simulink model "LKAS_AutoSave_DF_20220414_1924_SW62"  (R2018b)
settings: Solver=FixedStepDiscrete  StartTime=0.0  StopTime=10.0  FixedStep=0.01  RelTol=1e-3
model workspace (MAT data in the model file):
  MCOS : class17 (value not decoded)
  MCOS : class17 (value not decoded)
  MCOS : class17 (value not decoded)
  MCOS : class17 (value not decoded)
  MCOS : class17 (value not decoded)
  MCOS : class17 (value not decoded)
  MCOS : class17 (value not decoded)
  MCOS : class17 (value not decoded)
  MCOS : class17 (value not decoded)
  MCOS : class17 (value not decoded)
  MCOS : class17 (value not decoded)
  MCOS : class17 (value not decoded)
  MCOS : class17 (value not decoded)
  MCOS : class17 (value not decoded)
  MCOS : class17 (value not decoded)
  MCOS : class17 (value not decoded)
  MCOS : class17 (value not decoded)
  MCOS : class17 (value not decoded)
  MCOS : class17 (value not decoded)
  MCOS : class17 (value not decoded)
  MCOS : class17 (value not decoded)
  MCOS : class17 (value not decoded)
  MCOS : class17 (value not decoded)
  MCOS : class17 (value not decoded)
  MCOS : class17 (value not decoded)
  MCOS : class17 (value not decoded)
  MCOS : class17 (value not decoded)
  MCOS : class17 (value not decoded)
  MCOS : class17 (value not decoded)
  MCOS : class17 (value not decoded)
  MCOS : class17 (value not decoded)
  MCOS : class17 (value not decoded)
  MCOS : class17 (value not decoded)
  MCOS : class17 (value not decoded)
  MCOS : class17 (value not decoded)
  MCOS : class17 (value not decoded)
  MCOS : class17 (value not decoded)
  MCOS : class17 (value not decoded)
  MCOS : class17 (value not decoded)
  MCOS : class17 (value not decoded)
  MCOS : class17 (value not decoded)
  MCOS : class17 (value not decoded)
  MCOS : class17 (value not decoded)
  MCOS : class17 (value not decoded)
  MCOS : class17 (value not decoded)
  MCOS : class17 (value not decoded)
  MCOS : class17 (value not decoded)
  MCOS : class17 (value not decoded)
  MCOS : class17 (value not decoded)
  MCOS : class17 (value not decoded)
  MCOS : class17 (value not decoded)
  MCOS : class17 (value not decoded)
  MCOS : class17 (value not decoded)
  MCOS : class17 (value not decoded)
  MCOS : class17 (value not decoded)
  MCOS : class17 (value not decoded)
  MCOS : class17 (value not decoded)
  MCOS : class17 (value not decoded)
  MCOS : class17 (value not decoded)
  MCOS : class17 (value not decoded)
  MCOS : class17 (value not decoded)
  MCOS : class17 (value not decoded)
  MCOS : class17 (value not decoded)
  MCOS : class17 (value not decoded)
  MCOS : class17 (value not decoded)
  MCOS : class17 (value not decoded)
  MCOS : class17 (value not decoded)
  MCOS : class17 (value not decoded)
  MCOS : class17 (value not decoded)
  MCOS : class17 (value not decoded)
  MCOS : class17 (value not decoded)
  MCOS : class17 (value not decoded)
  MCOS : class17 (value not decoded)
  MCOS : class17 (value not decoded)
  MCOS : class17 (value not decoded)
  MCOS : class17 (value not decoded)
  MCOS : class17 (value not decoded)
  MCOS : class17 (value not decoded)
  MCOS : class17 (value not decoded)
  MCOS : class17 (value not decoded)
  MCOS : class17 (value not decoded)
  MCOS : class17 (value not decoded)
  MCOS : class17 (value not decoded)
  MCOS : class17 (value not decoded)
  MCOS : class17 (value not decoded)
  MCOS : class17 (value not decoded)
  MCOS : class17 (value not decoded)
  MCOS : class17 (value not decoded)
  MCOS : class17 (value not decoded)
  MCOS : class17 (value not decoded)
  MCOS : class17 (value not decoded)
  MCOS : class17 (value not decoded)
  MCOS : class17 (value not decoded)
  MCOS : class17 (value not decoded)
  MCOS : class17 (value not decoded)
  MCOS : class17 (value not decoded)
  MCOS : class17 (value not decoded)
  MCOS : class17 (value not decoded)
  MCOS : class17 (value not decoded)
  MCOS : class17 (value not decoded)
  MCOS : class17 (value not decoded)
  MCOS : class17 (value not decoded)
  MCOS : class17 (value not decoded)
  MCOS : class17 (value not decoded)
  MCOS : class17 (value not decoded)
  MCOS : class17 (value not decoded)
  MCOS : class17 (value not decoded)
  MCOS : class17 (value not decoded)
  MCOS : class17 (value not decoded)
undefined symbols (not defined in the file): LKA_CarWidth, LKA_SampleTime, LKA_StrRatio_C, LKA_Veh2CamL_C, LKA_Veh2CamW_C, LKA_WhlBaseL_C, LL_CompHdAg_C, LL_CompSWA_C, LL_CrvtPrvwT_C, LL_DesDvt_C, LL_DvtComp_C, LL_DvtPrvwT_C, LL_DvtSpdDet_vDvtSpdMin_C, LL_HandsOff_ExitTime, LL_HandsOff_TextTime, LL_HandsOff_WarnTime, LL_HdAgExT_C, LL_HdAgPrvwT_C, LL_LAccMax_C, LL_LAccRMax_C, LL_LDW_EarliestWarnLine_C, LL_LDW_LatestWarnLine_C, LL_LDWS_SUPPRESS_HEADING, LL_LFClb_TFC_FfCtlRatio_C, LL_LFClb_TFC_KdBalance_C, LL_LFClb_TFC_KdMaxSWA_C, LL_LFClb_TFC_KdV1_C, LL_LFClb_TFC_KdV2_C, LL_LFClb_TFC_KdVehSpdLwr_C, LL_LFClb_TFC_KdVehSpdUpr_C, LL_LFClb_TFC_Ki_C, LL_LFClb_TFC_KiMaxSWA_C, LL_LFClb_TFC_Kp_C, LL_LFClb_TFC_KpKlat_C, LL_LFClb_TFC_KpV1_C, LL_LFClb_TFC_KpV2_C, LL_LFClb_TFC_KpVehSpdLwr_C, LL_LFClb_TFC_KpVehSpdUpr_C, LL_LFClb_TFC_PrvwT_C, LL_LKA_EarliestWarnLine_C, LL_LKA_EnableLine_DvtMax, LL_LKA_EnableLine_DvtMin, LL_LKA_EnableLine_Max, LL_LKA_LatestWarnLine_C, LL_LKAExPrcs_ExitC0Dvt, LL_LKAExPrcs_ExitC0Swt, LL_LKAExPrcs_tiExitDelayTime3, LL_LKAExPrcs_tiExitTime1, LL_LKAExPrcs_tiExitTime2, LL_LKAExPrcs_tiExitTime3, LL_LKAS_OUT_OF_CONTROL_LAT_VEL, LL_LKAS_OUT_OF_CONTROL_TTLC, LL_LKASWASyn_M0, LL_LKASWASyn_M1, LL_LKASWASyn_M2, LL_LKASWASyn_M3D, LL_LKASWASyn_M3K_DT, LL_LKASWASyn_M3K_MSD, LL_LKASWASyn_M4K, LL_LKASWASyn_SWAaddMax ... (+50)
libraries: simulink x234, canmsglib x6, dspstat3 x3, simulink_extras x1
(part 5 of 17)

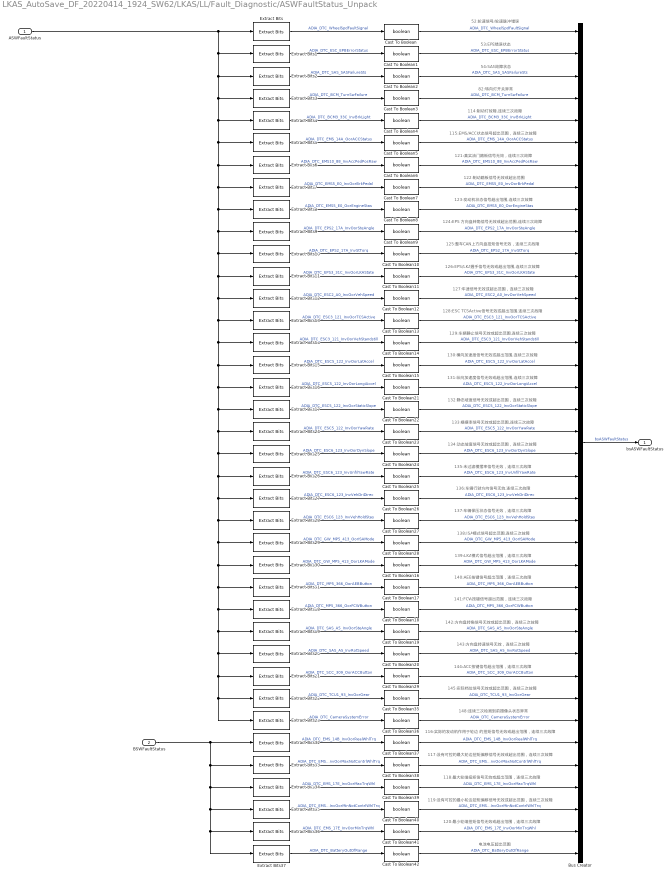
== system LKAS_AutoSave_DF_20220414_1924_SW62/LKAS/LL/Fault_Diagnostic/ASWFaultStatus_Unpack ==
  note: 117:没有可控的最大轮边扭矩偏移信号无效或超出范围，连续三次故障
  note: 120:最小轮端扭矩信号无效或超出范围，连续三次故障
  note: 116:实际的发动机作用于轮边 的扭矩信号无效或超出范围，连续三次故障
  note: 119:没有可控的最小轮边扭矩偏移信号无效或超出范围，连续三次故障
  note: 118:最大轮端扭矩信号无效或超出范围，连续三次故障
  note: 电池电压超出范围
  note: 148:连续三次检测到前摄像头状态异常
  note: 143:方向盘转速信号无效，连续三次故障
  note: 144:ACC按键信号超出范围，连续三次故障
  note: 145:实际档位信号无效或超出范围，连续三次故障
  note: 54:SAS故障状态
  note: 142:方向盘转角信号无效或超出范围，连续三次故障
  note: 121:真实油门踏板信号无效，连续三次故障
  note: 137:车辆保压状态信号无效，连续三次故障
  note: 114:制动灯故障,连续三次故障
  note: 115:EMS/ACC状态信号超出范围，连续三次故障
  note: 139:LKA模式信号超出范围，连续三次故障
  note: 53:EPB错误状态
  note: 123:发动机状态信号超出范围,连续三次故障
  note: 122:制动踏板信号无效或超出范围
  note: 124:EPS 方向盘转角信号无效或超出范围,连续三次故障
  note: 82:转向灯开关异常
  note: 52:轮速信号/轮速脉冲错误
  note: 130:横向加速度信号无效或超出范围,连续三次故障
  note: 134:动态坡度信号无效或超出范围，连续三次故障
  note: 131:纵向加速度信号无效或超出范围,连续三次故障
  note: 129:车辆静止信号无效或超出范围,连续三次故障
  note: 140:AEB按键信号超出范围，连续三次故障
  note: 128:ESC TCSActive信号无效或超出范围,连续三次故障
  note: 126:EPS/LKA握手信号无效或超出范围,连续三次故障
  note: 125:整车CAN上方向盘扭矩信号无效，连续三次故障
  note: 127:车速信号无效或超出范围，连续三次故障
  note: 141:FCW按键信号超出范围，连续三次故障
  note: 136:车辆行驶方向信号无效,连续三次故障
  note: 138:ISA模式信号超出范围,连续三次故障
  note: 135:未过滤横摆率信号无效，连续三次故障
  note: 133:横摆率信号无效或超出范围,连续三次故障
  note: 132:静态坡度信号无效或超出范围，连续三次故障
  ASWFaultStatus : Inport
  BSWFaultStatus : Inport  Port=2
  Bus Creator : BusCreator  Inputs=38
  Cast To Boolean{,1..29,35..42} (38 alike) : DataTypeConversion  OutDataTypeStr=boolean
  Extract Bits : simulink/Logic and Bit Operations/Extract Bits  bitsToExtract=Range of bits  numBits=8  bitIdxRange=0  outScalingMode=Preserve fixed-point scaling
      settings: SourceProductName=Simulink
  Extract Bits1 : simulink/Logic and Bit Operations/Extract Bits  bitsToExtract=Range of bits  numBits=8  bitIdxRange=1  outScalingMode=Treat bit field as an integer
      settings: SourceProductName=Simulink
  Extract Bits10 : simulink/Logic and Bit Operations/Extract Bits  bitsToExtract=Range of bits  numBits=8  bitIdxRange=10  outScalingMode=Treat bit field as an integer
      settings: SourceProductName=Simulink
  Extract Bits11 : simulink/Logic and Bit Operations/Extract Bits  bitsToExtract=Range of bits  numBits=8  bitIdxRange=11  outScalingMode=Treat bit field as an integer
      settings: SourceProductName=Simulink
  Extract Bits12 : simulink/Logic and Bit Operations/Extract Bits  bitsToExtract=Range of bits  numBits=8  bitIdxRange=12  outScalingMode=Treat bit field as an integer
      settings: SourceProductName=Simulink
  Extract Bits13 : simulink/Logic and Bit Operations/Extract Bits  bitsToExtract=Range of bits  numBits=8  bitIdxRange=13  outScalingMode=Treat bit field as an integer
      settings: SourceProductName=Simulink
  Extract Bits14 : simulink/Logic and Bit Operations/Extract Bits  bitsToExtract=Range of bits  numBits=8  bitIdxRange=14  outScalingMode=Treat bit field as an integer
      settings: SourceProductName=Simulink
  Extract Bits15 : simulink/Logic and Bit Operations/Extract Bits  bitsToExtract=Range of bits  numBits=8  bitIdxRange=15  outScalingMode=Treat bit field as an integer
      settings: SourceProductName=Simulink
  Extract Bits16 : simulink/Logic and Bit Operations/Extract Bits  bitsToExtract=Range of bits  numBits=8  bitIdxRange=16  outScalingMode=Treat bit field as an integer
      settings: SourceProductName=Simulink
  Extract Bits17 : simulink/Logic and Bit Operations/Extract Bits  bitsToExtract=Range of bits  numBits=8  bitIdxRange=17  outScalingMode=Treat bit field as an integer
      settings: SourceProductName=Simulink
  Extract Bits18 : simulink/Logic and Bit Operations/Extract Bits  bitsToExtract=Range of bits  numBits=8  bitIdxRange=26  outScalingMode=Treat bit field as an integer
      settings: SourceProductName=Simulink
  Extract Bits19 : simulink/Logic and Bit Operations/Extract Bits  bitsToExtract=Range of bits  numBits=8  bitIdxRange=27  outScalingMode=Treat bit field as an integer
      settings: SourceProductName=Simulink
  Extract Bits2 : simulink/Logic and Bit Operations/Extract Bits  bitsToExtract=Range of bits  numBits=8  bitIdxRange=2  outScalingMode=Treat bit field as an integer
      settings: SourceProductName=Simulink
  Extract Bits20 : simulink/Logic and Bit Operations/Extract Bits  bitsToExtract=Range of bits  numBits=8  bitIdxRange=28  outScalingMode=Treat bit field as an integer
      settings: SourceProductName=Simulink
  Extract Bits21 : simulink/Logic and Bit Operations/Extract Bits  bitsToExtract=Range of bits  numBits=8  bitIdxRange=29  outScalingMode=Treat bit field as an integer
      settings: SourceProductName=Simulink
  Extract Bits22 : simulink/Logic and Bit Operations/Extract Bits  bitsToExtract=Range of bits  numBits=8  bitIdxRange=30  outScalingMode=Treat bit field as an integer
      settings: SourceProductName=Simulink
  Extract Bits23 : simulink/Logic and Bit Operations/Extract Bits  bitsToExtract=Range of bits  numBits=8  bitIdxRange=31  outScalingMode=Treat bit field as an integer
      settings: SourceProductName=Simulink
  Extract Bits24 : simulink/Logic and Bit Operations/Extract Bits  bitsToExtract=Range of bits  numBits=8  bitIdxRange=18  outScalingMode=Treat bit field as an integer
      settings: SourceProductName=Simulink
  Extract Bits25 : simulink/Logic and Bit Operations/Extract Bits  bitsToExtract=Range of bits  numBits=8  bitIdxRange=19  outScalingMode=Treat bit field as an integer
      settings: SourceProductName=Simulink
  Extract Bits26 : simulink/Logic and Bit Operations/Extract Bits  bitsToExtract=Range of bits  numBits=8  bitIdxRange=20  outScalingMode=Treat bit field as an integer
      settings: SourceProductName=Simulink
  Extract Bits27 : simulink/Logic and Bit Operations/Extract Bits  bitsToExtract=Range of bits  numBits=8  bitIdxRange=21  outScalingMode=Treat bit field as an integer
      settings: SourceProductName=Simulink
  Extract Bits28 : simulink/Logic and Bit Operations/Extract Bits  bitsToExtract=Range of bits  numBits=8  bitIdxRange=22  outScalingMode=Treat bit field as an integer
      settings: SourceProductName=Simulink
  Extract Bits29 : simulink/Logic and Bit Operations/Extract Bits  bitsToExtract=Range of bits  numBits=8  bitIdxRange=23  outScalingMode=Treat bit field as an integer
      settings: SourceProductName=Simulink
  Extract Bits3 : simulink/Logic and Bit Operations/Extract Bits  bitsToExtract=Range of bits  numBits=8  bitIdxRange=3  outScalingMode=Treat bit field as an integer
      settings: SourceProductName=Simulink
  Extract Bits30 : simulink/Logic and Bit Operations/Extract Bits  bitsToExtract=Range of bits  numBits=8  bitIdxRange=24  outScalingMode=Treat bit field as an integer
      settings: SourceProductName=Simulink
  Extract Bits31 : simulink/Logic and Bit Operations/Extract Bits  bitsToExtract=Range of bits  numBits=8  bitIdxRange=25  outScalingMode=Treat bit field as an integer
      settings: SourceProductName=Simulink
  Extract Bits32 : simulink/Logic and Bit Operations/Extract Bits  bitsToExtract=Range of bits  numBits=8  bitIdxRange=26  outScalingMode=Treat bit field as an integer
      settings: SourceProductName=Simulink
  Extract Bits33 : simulink/Logic and Bit Operations/Extract Bits  bitsToExtract=Range of bits  numBits=8  bitIdxRange=27  outScalingMode=Treat bit field as an integer
      settings: SourceProductName=Simulink
  Extract Bits34 : simulink/Logic and Bit Operations/Extract Bits  bitsToExtract=Range of bits  numBits=8  bitIdxRange=28  outScalingMode=Treat bit field as an integer
      settings: SourceProductName=Simulink
  Extract Bits35 : simulink/Logic and Bit Operations/Extract Bits  bitsToExtract=Range of bits  numBits=8  bitIdxRange=29  outScalingMode=Treat bit field as an integer
      settings: SourceProductName=Simulink
  Extract Bits36 : simulink/Logic and Bit Operations/Extract Bits  bitsToExtract=Range of bits  numBits=8  bitIdxRange=30  outScalingMode=Treat bit field as an integer
      settings: SourceProductName=Simulink
  Extract Bits37 : simulink/Logic and Bit Operations/Extract Bits  bitsToExtract=Range of bits  numBits=8  bitIdxRange=31  outScalingMode=Treat bit field as an integer
      settings: SourceProductName=Simulink
  Extract Bits4 : simulink/Logic and Bit Operations/Extract Bits  bitsToExtract=Range of bits  numBits=8  bitIdxRange=4  outScalingMode=Treat bit field as an integer
      settings: SourceProductName=Simulink
  Extract Bits5 : simulink/Logic and Bit Operations/Extract Bits  bitsToExtract=Range of bits  numBits=8  bitIdxRange=5  outScalingMode=Treat bit field as an integer
      settings: SourceProductName=Simulink
  Extract Bits6 : simulink/Logic and Bit Operations/Extract Bits  bitsToExtract=Range of bits  numBits=8  bitIdxRange=6  outScalingMode=Treat bit field as an integer
      settings: SourceProductName=Simulink
  Extract Bits7 : simulink/Logic and Bit Operations/Extract Bits  bitsToExtract=Range of bits  numBits=8  bitIdxRange=7  outScalingMode=Treat bit field as an integer
      settings: SourceProductName=Simulink
  Extract Bits8 : simulink/Logic and Bit Operations/Extract Bits  bitsToExtract=Range of bits  numBits=8  bitIdxRange=8  outScalingMode=Treat bit field as an integer
      settings: SourceProductName=Simulink
  Extract Bits9 : simulink/Logic and Bit Operations/Extract Bits  bitsToExtract=Range of bits  numBits=8  bitIdxRange=9  outScalingMode=Treat bit field as an integer
      settings: SourceProductName=Simulink
  bsASWFaultStatus : Outport
  wires:
  Extract Bits37/1 -> Cast To Boolean42/1  "ADIA_DTC_BatteryOutOfRange"
  Extract Bits36/1 -> Cast To Boolean41/1  "ADIA_DTC_EMS_17E_InvOorMinTrqWhl"
  Extract Bits35/1 -> Cast To Boolean40/1  "ADIA_DTC_EMS_17E_InvOorMinNotContrlWhlTrq"
  Extract Bits34/1 -> Cast To Boolean39/1  "ADIA_DTC_EMS_17E_InvOorMaxTrqWhl"
  Extract Bits33/1 -> Cast To Boolean38/1  "ADIA_DTC_EMS_17E_InvOorMaxNotContrlWhlTrq"
  Extract Bits32/1 -> Cast To Boolean37/1  "ADIA_DTC_EMS_14B_InvOorRealWhlTrq"
  Extract Bits23/1 -> Cast To Boolean36/1  "ADIA_DTC_CameraSystemError"
  Extract Bits22/1 -> Cast To Boolean35/1  "ADIA_DTC_TCU1_93_InvOorGear"
  Extract Bits21/1 -> Cast To Boolean29/1  "ADIA_DTC_SCC_309_OorACCButton"
  Extract Bits20/1 -> Cast To Boolean20/1  "ADIA_DTC_SAS_A5_InvRotSpeed"
  Extract Bits19/1 -> Cast To Boolean19/1  "ADIA_DTC_SAS_A5_InvOorSteAngle"
  Extract Bits18/1 -> Cast To Boolean18/1  "ADIA_DTC_MP5_366_OorFCWButton"
  Extract Bits31/1 -> Cast To Boolean17/1  "ADIA_DTC_MP5_366_OorAEBButton"
  Extract Bits30/1 -> Cast To Boolean16/1  "ADIA_DTC_GW_MP5_413_OorLKAMode"
  Extract Bits29/1 -> Cast To Boolean28/1  "ADIA_DTC_GW_MP5_413_OorISAMode"
  Extract Bits28/1 -> Cast To Boolean27/1  "ADIA_DTC_ESC6_123_InvVehHoldStas"
  Extract Bits27/1 -> Cast To Boolean26/1  "ADIA_DTC_ESC6_123_InvVehDriDirec"
  Extract Bits26/1 -> Cast To Boolean25/1  "ADIA_DTC_ESC6_123_InvUnfilYawRate"
  Extract Bits25/1 -> Cast To Boolean24/1  "ADIA_DTC_ESC6_123_InvOorDynSlope"
  Extract Bits24/1 -> Cast To Boolean23/1  "ADIA_DTC_ESC5_122_InvOorYawRate"
  Extract Bits17/1 -> Cast To Boolean22/1  "ADIA_DTC_ESC5_122_InvOorStaticSlope"
  Extract Bits16/1 -> Cast To Boolean21/1  "ADIA_DTC_ESC5_122_InvOorLongiAccel"
  Extract Bits15/1 -> Cast To Boolean15/1  "ADIA_DTC_ESC5_122_InvOorLatAccel"
  Extract Bits14/1 -> Cast To Boolean14/1  "ADIA_DTC_ESC3_121_InvOorVehStandstill"
  Extract Bits13/1 -> Cast To Boolean13/1  "ADIA_DTC_ESC3_121_InvOorTCSActive"
  Extract Bits12/1 -> Cast To Boolean12/1  "ADIA_DTC_ESC2_A0_InvOorVehSpeed"
  Extract Bits11/1 -> Cast To Boolean11/1  "ADIA_DTC_EPS3_31C_InvOorLKAState"
  Extract Bits10/1 -> Cast To Boolean10/1  "ADIA_DTC_EPS2_17A_InvStTorq"
  Extract Bits9/1 -> Cast To Boolean9/1  "ADIA_DTC_EPS2_17A_InvOorSteAngle"
  Extract Bits8/1 -> Cast To Boolean8/1  "ADIA_DTC_EMS5_E0_OorEngineStas"
  Extract Bits7/1 -> Cast To Boolean7/1  "ADIA_DTC_EMS5_E0_InvOorBrkPedal"
  Extract Bits6/1 -> Cast To Boolean6/1  "ADIA_DTC_EMS10_88_InvAccPedPosRaw"
  Extract Bits5/1 -> Cast To Boolean5/1  "ADIA_DTC_EMS_14A_OorACCStatus"
  Extract Bits4/1 -> Cast To Boolean4/1  "ADIA_DTC_BCM3_33C_InvBrkLight"
  Extract Bits3/1 -> Cast To Boolean3/1  "ADIA_DTC_BCM_TurnSwFailure"
  Extract Bits2/1 -> Cast To Boolean2/1  "ADIA_DTC_SAS_SASFailureSts"
  Extract Bits1/1 -> Cast To Boolean1/1  "ADIA_DTC_ESC_EPBErrorStatus"
  Extract Bits/1 -> Cast To Boolean/1  "ADIA_DTC_WheelSpdFaultSignal"
  Cast To Boolean37/1 -> Bus Creator/33  "ADIA_DTC_EMS_14B_InvOorRealWhlTrq"
  BSWFaultStatus/1 -> Extract Bits37/1, Extract Bits36/1, Extract Bits35/1, Extract Bits34/1, Extract Bits33/1, Extract Bits32/1
  Cast To Boolean39/1 -> Bus Creator/35  "ADIA_DTC_EMS_17E_InvOorMaxTrqWhl"
  Cast To Boolean38/1 -> Bus Creator/34  "ADIA_DTC_EMS_17E_InvOorMaxNotContrlWhlTrq"
  Cast To Boolean40/1 -> Bus Creator/36  "ADIA_DTC_EMS_17E_InvOorMinNotContrlWhlTrq"
  Cast To Boolean41/1 -> Bus Creator/37  "ADIA_DTC_EMS_17E_InvOorMinTrqWhl"
  Cast To Boolean42/1 -> Bus Creator/38  "ADIA_DTC_BatteryOutOfRange"
  Cast To Boolean36/1 -> Bus Creator/32  "ADIA_DTC_CameraSystemError"
  Cast To Boolean29/1 -> Bus Creator/30  "ADIA_DTC_SCC_309_OorACCButton"
  Cast To Boolean16/1 -> Bus Creator/25  "ADIA_DTC_GW_MP5_413_OorLKAMode"
  Cast To Boolean20/1 -> Bus Creator/29  "ADIA_DTC_SAS_A5_InvRotSpeed"
  Cast To Boolean25/1 -> Bus Creator/21  "ADIA_DTC_ESC6_123_InvUnfilYawRate"
  Cast To Boolean24/1 -> Bus Creator/20  "ADIA_DTC_ESC6_123_InvOorDynSlope"
  Cast To Boolean21/1 -> Bus Creator/17  "ADIA_DTC_ESC5_122_InvOorLongiAccel"
  Cast To Boolean9/1 -> Bus Creator/10  "ADIA_DTC_EPS2_17A_InvOorSteAngle"
  Cast To Boolean6/1 -> Bus Creator/7  "ADIA_DTC_EMS10_88_InvAccPedPosRaw"
  Cast To Boolean7/1 -> Bus Creator/8  "ADIA_DTC_EMS5_E0_InvOorBrkPedal"
  Cast To Boolean3/1 -> Bus Creator/4  "ADIA_DTC_BCM_TurnSwFailure"
  Cast To Boolean4/1 -> Bus Creator/5  "ADIA_DTC_BCM3_33C_InvBrkLight"
  Cast To Boolean17/1 -> Bus Creator/26  "ADIA_DTC_MP5_366_OorAEBButton"
  Cast To Boolean27/1 -> Bus Creator/23  "ADIA_DTC_ESC6_123_InvVehHoldStas"
  Cast To Boolean8/1 -> Bus Creator/9  "ADIA_DTC_EMS5_E0_OorEngineStas"
  Cast To Boolean15/1 -> Bus Creator/16  "ADIA_DTC_ESC5_122_InvOorLatAccel"
  Bus Creator/1 -> bsASWFaultStatus/1  "bsASWFaultStatus"
  Cast To Boolean23/1 -> Bus Creator/19  "ADIA_DTC_ESC5_122_InvOorYawRate"
  Cast To Boolean/1 -> Bus Creator/1  "ADIA_DTC_WheelSpdFaultSignal"
  Cast To Boolean22/1 -> Bus Creator/18  "ADIA_DTC_ESC5_122_InvOorStaticSlope"
  Cast To Boolean18/1 -> Bus Creator/27  "ADIA_DTC_MP5_366_OorFCWButton"
  Cast To Boolean28/1 -> Bus Creator/24  "ADIA_DTC_GW_MP5_413_OorISAMode"
  Cast To Boolean12/1 -> Bus Creator/13  "ADIA_DTC_ESC2_A0_InvOorVehSpeed"
  Cast To Boolean11/1 -> Bus Creator/12  "ADIA_DTC_EPS3_31C_InvOorLKAState"
  Cast To Boolean10/1 -> Bus Creator/11  "ADIA_DTC_EPS2_17A_InvStTorq"
  Cast To Boolean14/1 -> Bus Creator/15  "ADIA_DTC_ESC3_121_InvOorVehStandstill"
  Cast To Boolean5/1 -> Bus Creator/6  "ADIA_DTC_EMS_14A_OorACCStatus"
  Cast To Boolean26/1 -> Bus Creator/22  "ADIA_DTC_ESC6_123_InvVehDriDirec"
  Cast To Boolean19/1 -> Bus Creator/28  "ADIA_DTC_SAS_A5_InvOorSteAngle"
  Cast To Boolean13/1 -> Bus Creator/14  "ADIA_DTC_ESC3_121_InvOorTCSActive"
  Cast To Boolean1/1 -> Bus Creator/2  "ADIA_DTC_ESC_EPBErrorStatus"
  Cast To Boolean2/1 -> Bus Creator/3  "ADIA_DTC_SAS_SASFailureSts"
  Cast To Boolean35/1 -> Bus Creator/31  "ADIA_DTC_TCU1_93_InvOorGear"
  ASWFaultStatus/1 -> Extract Bits23/1, Extract Bits22/1, Extract Bits21/1, Extract Bits20/1, Extract Bits19/1, Extract Bits18/1, Extract Bits31/1, Extract Bits30/1, Extract Bits29/1, Extract Bits28/1, Extract Bits27/1, Extract Bits26/1, Extract Bits25/1, Extract Bits24/1, Extract Bits17/1, Extract Bits16/1, Extract Bits15/1, Extract Bits14/1, Extract Bits13/1, Extract Bits12/1, Extract Bits11/1, Extract Bits10/1, Extract Bits9/1, Extract Bits8/1, Extract Bits7/1, Extract Bits6/1, Extract Bits5/1, Extract Bits4/1, Extract Bits3/1, Extract Bits2/1, Extract Bits1/1, Extract Bits/1

== system LKAS_AutoSave_DF_20220414_1924_SW62/LKAS/LL/Fault_Diagnostic/BSWFaultStatus_Unpack ==
  note: 角雷达故障
  note: 前雷达内部故障
  note: EPB节点通信丢失
  note: ACU节点通信丢失
  note: BCM节点通信丢失
  note: SAS节点通信丢失
  note: ESC节点通信丢失
  note: EMS节点通信丢失
  note: IC节点通信丢失
  note: MP5节点通信丢失
  note: TBox节点通信丢失
  note: TCU节点通信丢失
  note: EPS节点通信丢失
  BSWFaultStatus : Inport
  Bus Creator : BusCreator  Inputs=13
  Cast To Boolean{,1..12} (13 alike) : DataTypeConversion  OutDataTypeStr=boolean
  Extract Bits : simulink/Logic and Bit Operations/Extract Bits  bitsToExtract=Range of bits  numBits=8  bitIdxRange=0  outScalingMode=Treat bit field as an integer
      settings: SourceProductName=Simulink
  Extract Bits1 : simulink/Logic and Bit Operations/Extract Bits  bitsToExtract=Range of bits  numBits=8  bitIdxRange=1  outScalingMode=Treat bit field as an integer
      settings: SourceProductName=Simulink
  Extract Bits10 : simulink/Logic and Bit Operations/Extract Bits  bitsToExtract=Range of bits  numBits=8  bitIdxRange=10  outScalingMode=Treat bit field as an integer
      settings: SourceProductName=Simulink
  Extract Bits16 : simulink/Logic and Bit Operations/Extract Bits  bitsToExtract=Range of bits  numBits=8  bitIdxRange=16  outScalingMode=Treat bit field as an integer
      settings: SourceProductName=Simulink
  Extract Bits17 : simulink/Logic and Bit Operations/Extract Bits  bitsToExtract=Range of bits  numBits=8  bitIdxRange=17  outScalingMode=Treat bit field as an integer
      settings: SourceProductName=Simulink
  Extract Bits2 : simulink/Logic and Bit Operations/Extract Bits  bitsToExtract=Range of bits  numBits=8  bitIdxRange=2  outScalingMode=Treat bit field as an integer
      settings: SourceProductName=Simulink
  Extract Bits3 : simulink/Logic and Bit Operations/Extract Bits  bitsToExtract=Range of bits  numBits=8  bitIdxRange=3  outScalingMode=Treat bit field as an integer
      settings: SourceProductName=Simulink
  Extract Bits4 : simulink/Logic and Bit Operations/Extract Bits  bitsToExtract=Range of bits  numBits=8  bitIdxRange=4  outScalingMode=Treat bit field as an integer
      settings: SourceProductName=Simulink
  Extract Bits5 : simulink/Logic and Bit Operations/Extract Bits  bitsToExtract=Range of bits  numBits=8  bitIdxRange=5  outScalingMode=Treat bit field as an integer
      settings: SourceProductName=Simulink
  Extract Bits6 : simulink/Logic and Bit Operations/Extract Bits  bitsToExtract=Range of bits  numBits=8  bitIdxRange=6  outScalingMode=Treat bit field as an integer
      settings: SourceProductName=Simulink
  Extract Bits7 : simulink/Logic and Bit Operations/Extract Bits  bitsToExtract=Range of bits  numBits=8  bitIdxRange=7  outScalingMode=Treat bit field as an integer
      settings: SourceProductName=Simulink
  Extract Bits8 : simulink/Logic and Bit Operations/Extract Bits  bitsToExtract=Range of bits  numBits=8  bitIdxRange=8  outScalingMode=Treat bit field as an integer
      settings: SourceProductName=Simulink
  Extract Bits9 : simulink/Logic and Bit Operations/Extract Bits  bitsToExtract=Range of bits  numBits=8  bitIdxRange=9  outScalingMode=Treat bit field as an integer
      settings: SourceProductName=Simulink
  bsBSWFaultStatus : Outport
  wires:
  Extract Bits17/1 -> Cast To Boolean12/1  "ADIAve_d_sen_sta_Corner_radar"
  Extract Bits16/1 -> Cast To Boolean11/1  "ADIA_Inner_FRadar_FaultState"
  Extract Bits10/1 -> Cast To Boolean10/1  "ADIAve_e_Node_EPB_Validity"
  Extract Bits9/1 -> Cast To Boolean9/1  "ADIAve_e_Node_TCU_Validity"
  Extract Bits8/1 -> Cast To Boolean8/1  "ADIAve_e_Node_MP5_Validity"
  Extract Bits7/1 -> Cast To Boolean7/1  "ADIAve_e_Node_TBOX_Validity"
  Extract Bits6/1 -> Cast To Boolean6/1  "ADIAve_e_Node_IC_Validity"
  Extract Bits5/1 -> Cast To Boolean5/1  "ADIAve_e_Node_EMS_Validity"
  Extract Bits4/1 -> Cast To Boolean4/1  "ADIAve_e_Node_SAS_Validity"
  Extract Bits3/1 -> Cast To Boolean3/1  "ADIAve_e_Node_IBCM_Validity"
  Extract Bits2/1 -> Cast To Boolean2/1  "ADIAve_e_Node_ESC_Validity"
  Extract Bits1/1 -> Cast To Boolean1/1  "ADIAve_e_Node_EPS_Validity"
  Extract Bits/1 -> Cast To Boolean/1  "ADIAve_e_Node_ACU_Validity"
  BSWFaultStatus/1 -> Extract Bits16/1, Extract Bits17/1, Extract Bits10/1, Extract Bits9/1, Extract Bits8/1, Extract Bits7/1, Extract Bits6/1, Extract Bits5/1, Extract Bits4/1, Extract Bits3/1, Extract Bits2/1, Extract Bits1/1, Extract Bits/1
  Cast To Boolean2/1 -> Bus Creator/3  "ADIAve_e_Node_ESC_Validity"
  Cast To Boolean1/1 -> Bus Creator/2  "ADIAve_e_Node_EPS_Validity"
  Cast To Boolean5/1 -> Bus Creator/6  "ADIAve_e_Node_EMS_Validity"
  Cast To Boolean10/1 -> Bus Creator/11  "ADIAve_e_Node_EPB_Validity"
  Cast To Boolean12/1 -> Bus Creator/13  "ADIAve_d_sen_sta_Corner_radar"
  Cast To Boolean/1 -> Bus Creator/1  "ADIAve_e_Node_ACU_Validity"
  Bus Creator/1 -> bsBSWFaultStatus/1  "bsBSWFaultStatus"
  Cast To Boolean8/1 -> Bus Creator/9  "ADIAve_e_Node_MP5_Validity"
  Cast To Boolean4/1 -> Bus Creator/5  "ADIAve_e_Node_SAS_Validity"
  Cast To Boolean3/1 -> Bus Creator/4  "ADIAve_e_Node_IBCM_Validity"
  Cast To Boolean7/1 -> Bus Creator/8  "ADIAve_e_Node_TBOX_Validity"
  Cast To Boolean6/1 -> Bus Creator/7  "ADIAve_e_Node_IC_Validity"
  Cast To Boolean9/1 -> Bus Creator/10  "ADIAve_e_Node_TCU_Validity"
  Cast To Boolean11/1 -> Bus Creator/12  "ADIA_Inner_FRadar_FaultState"

== system LKAS_AutoSave_DF_20220414_1924_SW62/LKAS/LL/Fault_Diagnostic/FuncFaultStatus_Unpack ==
  note: ob_ADIA_SpareDataCheck
  FuncFaultStatus : Inport
  Bus Creator : BusCreator  Inputs=16
  Extract Bits : simulink/Logic and Bit Operations/Extract Bits  bitsToExtract=Range of bits  numBits=8  bitIdxRange=0  outScalingMode=Treat bit field as an integer
      settings: SourceProductName=Simulink
  Extract Bits1 : simulink/Logic and Bit Operations/Extract Bits  bitsToExtract=Range of bits  numBits=8  bitIdxRange=1  outScalingMode=Treat bit field as an integer
      settings: SourceProductName=Simulink
  Extract Bits10 : simulink/Logic and Bit Operations/Extract Bits  bitsToExtract=Range of bits  numBits=8  bitIdxRange=10  outScalingMode=Treat bit field as an integer
      settings: SourceProductName=Simulink
  Extract Bits11 : simulink/Logic and Bit Operations/Extract Bits  bitsToExtract=Range of bits  numBits=8  bitIdxRange=11  outScalingMode=Treat bit field as an integer
      settings: SourceProductName=Simulink
  Extract Bits12 : simulink/Logic and Bit Operations/Extract Bits  bitsToExtract=Range of bits  numBits=8  bitIdxRange=12  outScalingMode=Treat bit field as an integer
      settings: SourceProductName=Simulink
  Extract Bits13 : simulink/Logic and Bit Operations/Extract Bits  bitsToExtract=Range of bits  numBits=8  bitIdxRange=13  outScalingMode=Treat bit field as an integer
      settings: SourceProductName=Simulink
  Extract Bits14 : simulink/Logic and Bit Operations/Extract Bits  bitsToExtract=Range of bits  numBits=8  bitIdxRange=14  outScalingMode=Treat bit field as an integer
      settings: SourceProductName=Simulink
  Extract Bits15 : simulink/Logic and Bit Operations/Extract Bits  bitsToExtract=Range of bits  numBits=8  bitIdxRange=15  outScalingMode=Treat bit field as an integer
      settings: SourceProductName=Simulink
  Extract Bits2 : simulink/Logic and Bit Operations/Extract Bits  bitsToExtract=Range of bits  numBits=8  bitIdxRange=2  outScalingMode=Treat bit field as an integer
      settings: SourceProductName=Simulink
  Extract Bits3 : simulink/Logic and Bit Operations/Extract Bits  bitsToExtract=Range of bits  numBits=8  bitIdxRange=3  outScalingMode=Treat bit field as an integer
      settings: SourceProductName=Simulink
  Extract Bits4 : simulink/Logic and Bit Operations/Extract Bits  bitsToExtract=Range of bits  numBits=8  bitIdxRange=4  outScalingMode=Treat bit field as an integer
      settings: SourceProductName=Simulink
  Extract Bits5 : simulink/Logic and Bit Operations/Extract Bits  bitsToExtract=Range of bits  numBits=8  bitIdxRange=5  outScalingMode=Treat bit field as an integer
      settings: SourceProductName=Simulink
  Extract Bits6 : simulink/Logic and Bit Operations/Extract Bits  bitsToExtract=Range of bits  numBits=8  bitIdxRange=6  outScalingMode=Treat bit field as an integer
      settings: SourceProductName=Simulink
  Extract Bits7 : simulink/Logic and Bit Operations/Extract Bits  bitsToExtract=Range of bits  numBits=8  bitIdxRange=7  outScalingMode=Treat bit field as an integer
      settings: SourceProductName=Simulink
  Extract Bits8 : simulink/Logic and Bit Operations/Extract Bits  bitsToExtract=Range of bits  numBits=8  bitIdxRange=8  outScalingMode=Treat bit field as an integer
      settings: SourceProductName=Simulink
  Extract Bits9 : simulink/Logic and Bit Operations/Extract Bits  bitsToExtract=Range of bits  numBits=8  bitIdxRange=9  outScalingMode=Treat bit field as an integer
      settings: SourceProductName=Simulink
  bsFuncFaultStatus : Outport
  wires:
  Extract Bits9/1 -> Bus Creator/10
  Extract Bits6/1 -> Bus Creator/7
  Extract Bits7/1 -> Bus Creator/8
  Extract Bits3/1 -> Bus Creator/4
  Extract Bits4/1 -> Bus Creator/5
  Extract Bits8/1 -> Bus Creator/9  "ob_ADIA_SpareDataCheck"
  Extract Bits15/1 -> Bus Creator/16  "ob_DTC_AEB_Safety_Violation"
  Bus Creator/1 -> bsFuncFaultStatus/1  "bsFuncFaultStatus"
  Extract Bits/1 -> Bus Creator/1
  Extract Bits12/1 -> Bus Creator/13  "ob_DTC_ACC_Mixed_Mode_Conflict"
  Extract Bits11/1 -> Bus Creator/12  "ob_DTC_ACC_Accel_Decel_Safety_Violation"
  Extract Bits10/1 -> Bus Creator/11
  Extract Bits14/1 -> Bus Creator/15  "ob_DTC_ACC_HoldConfirm_Safety_Violation"
  Extract Bits5/1 -> Bus Creator/6
  Extract Bits13/1 -> Bus Creator/14  "ob_DTC_ACC_Displacement_Safety_Violation"
  Extract Bits1/1 -> Bus Creator/2
  Extract Bits2/1 -> Bus Creator/3
  FuncFaultStatus/1 -> Extract Bits15/1, Extract Bits14/1, Extract Bits13/1, Extract Bits12/1, Extract Bits11/1, Extract Bits10/1, Extract Bits9/1, Extract Bits8/1, Extract Bits7/1, Extract Bits6/1, Extract Bits5/1, Extract Bits4/1, Extract Bits3/1, Extract Bits2/1, Extract Bits1/1, Extract Bits/1

== system LKAS_AutoSave_DF_20220414_1924_SW62/LKAS/LL/Human Machine Interface (HMI)/Subsystem ==
  LDW_State : Inport
  LKA_State : Inport  Port=2
  bsEPSInfo : Inport  Port=3
  LKA_SampleTime : Inport  Port=4
  LL_HandsOff_TextTime : Inport  Port=5
  LL_HandsOff_WarnTime : Inport  Port=6
  LL_RlsDet_tiTrqChkT_DISABLE : Inport  Port=7
  LL_RlsDet_tiTrqChkT_EPS_DISABLE : Inport  Port=8
  Abs : Abs
  Bus Selector2 : BusSelector  OutputSignals=EPS_LKA_State,EPS_SW_Trq
  Compare{1..2,4,7} (4 alike) : simulink/Logic and Bit Operations/Compare To Constant  relop===  const=3  OutDataTypeStr=boolean
  Compare3 : simulink/Logic and Bit Operations/Compare To Constant  relop===  const=1  OutDataTypeStr=boolean
  Compare5 : simulink/Logic and Bit Operations/Compare To Constant  relop===  const=4  OutDataTypeStr=boolean
  Compare6 : simulink/Logic and Bit Operations/Compare To Constant  relop===  const=5  OutDataTypeStr=boolean
  Compare8 : simulink/Logic and Bit Operations/Compare To Constant  relop===  const=4  OutDataTypeStr=boolean
  Compare9 : simulink/Logic and Bit Operations/Compare To Constant  relop===  const=5  OutDataTypeStr=boolean
  Logical Operator1 : Logic  Operator=OR  AllPortsSameDT=off  OutDataTypeStr=boolean
  Logical Operator2 : Logic  Inputs=3  AllPortsSameDT=off  OutDataTypeStr=boolean
  Logical Operator3 : Logic  Operator=OR  Inputs=6  AllPortsSameDT=off  OutDataTypeStr=boolean
  Relational Operator : RelationalOperator  Operator=<=  OutDataTypeStr=boolean  RndMeth=Nearest
  Sum Condition1 : Subsystem  TreatAsAtomicUnit=on
  Sum Condition2 : Subsystem  TreatAsAtomicUnit=on
  Switch : Switch  Criteria=u2 > Threshold
  HandsOff2_Warn : Outport
  HandsOff1_Text : Outport  Port=2
  wires:
  LKA_SampleTime/1 -> [LKA_SampleTime]
  Bus Selector2/2 -> Abs/1  "<EPS_SW_Trq>"
  LL_HandsOff_WarnTime/1 -> Sum Condition2/2(Sum)
  LL_HandsOff_TextTime/1 -> Sum Condition1/2(Sum)
  [LKA_SampleTime] -> Sum Condition2/1(SampleTime), Sum Condition1/1(SampleTime)
  Logical Operator1/1 -> Logical Operator2/2
  Compare3/1 -> Logical Operator1/2
  Compare2/1 -> Logical Operator1/1
  Compare7/1 -> Logical Operator3/6
  Compare8/1 -> Logical Operator3/5
  Compare9/1 -> Logical Operator3/4
  LKA_State/1 -> Compare7/1, Compare8/1, Compare9/1
  Abs/1 -> Relational Operator/1
  Compare6/1 -> Logical Operator3/1
  Compare5/1 -> Logical Operator3/2
  Compare4/1 -> Logical Operator3/3
  LDW_State/1 -> Compare5/1, Compare6/1, Compare4/1
  Sum Condition2/1(Out) -> HandsOff2_Warn/1
  Relational Operator/1 -> Logical Operator2/3
  LL_RlsDet_tiTrqChkT_DISABLE/1 -> Switch/3
  Logical Operator3/1 -> Logical Operator2/1
  Logical Operator2/1 -> Sum Condition1/Enable, Sum Condition2/Enable
  Compare1/1 -> Switch/2
  Switch/1 -> Relational Operator/2
  bsEPSInfo/1 -> Bus Selector2/1
  LL_RlsDet_tiTrqChkT_EPS_DISABLE/1 -> Switch/1
  Bus Selector2/1 -> Compare1/1, Compare2/1, Compare3/1  "<EPS_LKA_State>"
  Sum Condition1/1(Out) -> HandsOff1_Text/1

== system LKAS_AutoSave_DF_20220414_1924_SW62/LKAS/LL/LL Inputs Mapping/bsBCMInfo ==
  bsBCMInfoIn : Inport
  Bus Creator1 : BusCreator  Inputs=3
  Bus Selector1 : BusSelector  OutputSignals=BCM_Double_Light,BCM_Left_Light,BCM_Right_Light,BCM_LeftTurn_Switch,BCM_RightTurn_Switch
  Compare To Constant : simulink/Logic and Bit Operations/Compare To Constant  relop===  const=1  OutDataTypeStr=boolean
  Compare To Constant1 : simulink/Logic and Bit Operations/Compare To Constant  relop===  const=1  OutDataTypeStr=boolean
  Logical Operator : Logic  Operator=OR  AllPortsSameDT=off  OutDataTypeStr=boolean
  Logical Operator1 : Logic  Operator=OR  AllPortsSameDT=off  OutDataTypeStr=boolean
  bsBCMInfoOut : Outport
  wires:
  Logical Operator1/1 -> Bus Creator1/3  "BCM_Right_Light"
  Logical Operator/1 -> Bus Creator1/2  "BCM_Left_Light"
  Compare To Constant1/1 -> Logical Operator1/2
  Compare To Constant/1 -> Logical Operator/2
  Bus Selector1/5 -> Compare To Constant1/1  "<BCM_RightTurn_Switch>"
  Bus Selector1/4 -> Compare To Constant/1  "<BCM_LeftTurn_Switch>"
  bsBCMInfoIn/1 -> Bus Selector1/1
  Bus Selector1/1 -> Bus Creator1/1  "<BCM_Double_Light>"
  Bus Creator1/1 -> bsBCMInfoOut/1
  Bus Selector1/2 -> Logical Operator/1  "<BCM_Left_Light>"
  Bus Selector1/3 -> Logical Operator1/1  "<BCM_Right_Light>"

== system LKAS_AutoSave_DF_20220414_1924_SW62/LKAS/LL/LL Inputs Mapping/bsEPSInfo ==
  bsEPSInfoIn : Inport
  Bus Creator4 : BusCreator  Inputs=11
  Bus Selector1 : BusSelector  OutputSignals=EPS_LKA_State,EPS_SW_Trq,EPS_Trq_State,SAS_Clb_State,SAS_Trim_State,SWS_Failure_Status,EPS_TrqLim_State,EPS_LKA_Current,EPS_SWHold_State,EPS_Driver_Override,EPS_ESA_State
  bsEPSInfoOut : Outport
  wires:
  Bus Selector1/11 -> Bus Creator4/11  "<EPS_ESA_State>"
  Bus Selector1/10 -> Bus Creator4/10  "<EPS_Driver_Override>"
  Bus Selector1/6 -> Bus Creator4/6  "<SWS_Failure_Status>"
  bsEPSInfoIn/1 -> Bus Selector1/1
  Bus Selector1/2 -> Bus Creator4/2  "<EPS_SW_Trq>"
  Bus Selector1/1 -> Bus Creator4/1  "<EPS_LKA_State>"
  Bus Creator4/1 -> bsEPSInfoOut/1
  Bus Selector1/3 -> Bus Creator4/3  "<EPS_Trq_State>"
  Bus Selector1/4 -> Bus Creator4/4  "<SAS_Clb_State>"
  Bus Selector1/5 -> Bus Creator4/5  "<SAS_Trim_State>"
  Bus Selector1/7 -> Bus Creator4/7  "<EPS_TrqLim_State>"
  Bus Selector1/8 -> Bus Creator4/8  "<EPS_LKA_Current>"
  Bus Selector1/9 -> Bus Creator4/9  "<EPS_SWHold_State>"

== system LKAS_AutoSave_DF_20220414_1924_SW62/LKAS/LL/LL Inputs Mapping/bsLaneInfo ==
  bsLLClb : Inport
  bsLaneInfoIn : Inport  Port=2
  Bus Creator : BusCreator  Inputs=5
  Bus Selector1 : BusSelector  OutputSignals=bsFusL0Info,bsFusR0Info,bsFusL1Info,bsFusR1Info,bsFusLrgInfo,bsFusRrgInfo,Fusion_AdditionalInf
  LaneSelect : Subsystem
  "LanesReconstruct " : Subsystem
  bsLaneInfoOut : Outport
  wires:
  LaneSelect/6(bsRrgInfo) -> "LanesReconstruct "/7(bsRrgInfo)
  LaneSelect/5(bsLrgInfo) -> "LanesReconstruct "/6(bsLrgInfo)
  Bus Selector1/6 -> LaneSelect/6(bsFusRrgInfo)  "<bsFusRrgInfo>"
  Bus Selector1/5 -> LaneSelect/5(bsFusLrgInfo)  "<bsFusLrgInfo>"
  bsLLClb/1 -> "LanesReconstruct "/1(bsLLClb)
  bsLaneInfoIn/1 -> Bus Selector1/1
  Bus Selector1/7 -> Bus Creator/5  "<Fusion_AdditionalInf>"
  "LanesReconstruct "/1(bsL0InfoR) -> Bus Creator/1  "bsL0Info"
  "LanesReconstruct "/2(bsR0InfoR) -> Bus Creator/2  "bsR0Info"
  "LanesReconstruct "/3(bsL1InfoR) -> Bus Creator/3  "bsL1Info"
  "LanesReconstruct "/4(bsR1InfoR) -> Bus Creator/4  "bsR1Info"
  LaneSelect/1(bsL0Info) -> "LanesReconstruct "/2(bsL0Info)
  LaneSelect/2(bsR0Info) -> "LanesReconstruct "/3(bsR0Info)
  LaneSelect/3(bsL1Info) -> "LanesReconstruct "/4(bsL1Info)
  LaneSelect/4(bsR1Info) -> "LanesReconstruct "/5(bsR1Info)
  Bus Selector1/1 -> LaneSelect/1(bsFusL0Info)  "<bsFusL0Info>"
  Bus Selector1/2 -> LaneSelect/2(bsFusR0Info)  "<bsFusR0Info>"
  Bus Selector1/3 -> LaneSelect/3(bsFusL1Info)  "<bsFusL1Info>"
  Bus Selector1/4 -> LaneSelect/4(bsFusR1Info)  "<bsFusR1Info>"
  Bus Creator/1 -> bsLaneInfoOut/1

== system LKAS_AutoSave_DF_20220414_1924_SW62/LKAS/LL/LL Inputs Mapping/bsMP5Info ==
  note: ELK_Mode
      | 0: off
      | 1: LDW
      | 2: ~
      | 3: ELK
  note: LKA_Mode
      | 0: off
      | 1: LDW
      | 2: LKA
  note: LKA_Mode
      | 0: LDW
      | 1: LKA
      | 2: ~
  note: LkaFcnConf
      | 0: OFF
      | 1: LDW-声音
      | 2: LDW-振动
      | 3: LDW-声音+振动
      | 4: LKA-声音
      | 5: LKA-振动
      | 6: LKA-声音+振动
      | 7: LDW-声音-ICA
      | 8: LDW-振动-ICA
      | 9: LDW-声音+振动-ICA
      | 10: LKA-声音-ICA
      | 11: LKA-振动-ICA
      | 12: LKA-声音+振动-ICA
  note: LDW_Warn_Mode
      | 0: 声音
      | 1: 振动
      | 2: 声音+振动
  bsMP5InfoIn : Inport
  Bus Creator : BusCreator  Inputs=6
  Bus Selector1 : BusSelector  OutputSignals=LkaFcnConf,LKA_Main_Switch,LKA_Mode,LDW_Warn_Mode,APA_AutoPark_WorkSt,MP5_Work_State
  Cast To Boolean : DataTypeConversion  OutDataTypeStr=boolean
  MATLAB Function : MATLAB Function  TreatAsAtomicUnit=on
  bsMP5InfoOut : Outport
  wires:
  Cast To Boolean/1 -> MATLAB Function/2(LKA_Main_Switch_In)
  MATLAB Function/2(LKA_Switch) -> Bus Creator/2  "LKA_Switch"
  Bus Selector1/2 -> Cast To Boolean/1  "<LKA_Main_Switch>"
  Bus Selector1/1 -> MATLAB Function/1(LkaFcnConf)  "<LkaFcnConf>"
  MATLAB Function/1(LKA_Main_Switch) -> Bus Creator/1  "LKA_Main_Switch"
  MATLAB Function/4(LDW_Warn_Mode) -> Bus Creator/4  "LDW_Warn_Mode"
  MATLAB Function/3(LKA_Mode) -> Bus Creator/3  "LKA_Mode"
  Bus Selector1/4 -> MATLAB Function/4(LDW_Warn_Mode_In)  "<LDW_Warn_Mode>"
  Bus Selector1/3 -> MATLAB Function/3(LKA_Mode_In)  "<LKA_Mode>"
  Bus Creator/1 -> bsMP5InfoOut/1
  Bus Selector1/6 -> Bus Creator/6  "<MP5_Work_State>"
  Bus Selector1/5 -> Bus Creator/5  "<APA_AutoPark_WorkSt>"
  bsMP5InfoIn/1 -> Bus Selector1/1

== system LKAS_AutoSave_DF_20220414_1924_SW62/LKAS/LL/LL Inputs Mapping/bsPTState ==
  bsPTStateIn : Inport
  Bus Creator3 : BusCreator  Inputs=3
  Bus Selector1 : BusSelector  OutputSignals=AccPedal_Pos,TCU_ActualGear,TCU_Available
  Constant1 : Constant  Value=0  OutDataTypeStr=uint8
  Constant3 : Constant  Value=3  OutDataTypeStr=uint8
  Multiport Switch : MultiPortSwitch  DataPortOrder=Zero-based contiguous  Inputs=11  zeroidx=on
  bsPTStateOut : Outport
  wires:
  Bus Selector1/3 -> Bus Creator3/3  "<TCU_Available>"
  Constant1/1 -> Multiport Switch/2, Multiport Switch/7, Multiport Switch/8, Multiport Switch/12
  Bus Selector1/2 -> Multiport Switch/1  "<TCU_ActualGear>"
  Constant3/1 -> Multiport Switch/3, Multiport Switch/4, Multiport Switch/5, Multiport Switch/6, Multiport Switch/9, Multiport Switch/10, Multiport Switch/11
  Multiport Switch/1 -> Bus Creator3/2  "TCU_ActualGear"
  bsPTStateIn/1 -> Bus Selector1/1
  Bus Selector1/1 -> Bus Creator3/1  "<AccPedal_Pos>"
  Bus Creator3/1 -> bsPTStateOut/1

== system LKAS_AutoSave_DF_20220414_1924_SW62/LKAS/LL/LL Inputs Mapping/bsSWAInfo ==
  bsSWAInfoIn : Inport
  Bus Creator : BusCreator  Inputs=4
  Bus Selector1 : BusSelector  OutputSignals=EPS_SteeringAngle_Flag,EPS_SteeringAngle,SW_Angle,SW_Angle_Speed
  Gain : Gain
  bsSWAInfoOut : Outport
  wires:
  Bus Selector1/1 -> Bus Creator/1  "<EPS_SteeringAngle_Flag>"
  Bus Selector1/2 -> Gain/1, Bus Creator/2  "<EPS_SteeringAngle>"
  bsSWAInfoIn/1 -> Bus Selector1/1
  Gain/1 -> Bus Creator/3  "SW_Angle"
  Bus Selector1/4 -> Bus Creator/4  "<SW_Angle_Speed>"
  Bus Creator/1 -> bsSWAInfoOut/1

== system LKAS_AutoSave_DF_20220414_1924_SW62/LKAS/LL/LL Inputs Mapping/bsVehMovInfo ==
  bsVehMovInfoIn : Inport
  Bus Creator : BusCreator  Inputs=10
  Bus Selector2 : BusSelector  OutputSignals=ESC_LatAcc,ESC_LatAcc_Valid,ESC_YawRate,ESC_YawRate_Valid,ESC_UnYawRate,ESC_VehSpd,ESC_LonAcc,ESC_LonAcc_Valid,ESC_Brake_Press,ESC_VehSpd_Valid
  Saturation : Saturate  UpperLimit=inf  LowerLimit=0.1
  bsVehMovInfoOut : Outport
  wires:
  Saturation/1 -> Bus Creator/6  "ESC_VehSpd"
  bsVehMovInfoIn/1 -> Bus Selector2/1
  Bus Selector2/1 -> Bus Creator/1  "<ESC_LatAcc>"
  Bus Selector2/2 -> Bus Creator/2  "<ESC_LatAcc_Valid>"
  Bus Selector2/3 -> Bus Creator/3  "<ESC_YawRate>"
  Bus Selector2/4 -> Bus Creator/4  "<ESC_YawRate_Valid>"
  Bus Selector2/5 -> Bus Creator/5  "<ESC_UnYawRate>"
  Bus Selector2/6 -> Saturation/1  "<ESC_VehSpd>"
  Bus Selector2/7 -> Bus Creator/7  "<ESC_LonAcc>"
  Bus Selector2/8 -> Bus Creator/8  "<ESC_LonAcc_Valid>"
  Bus Selector2/9 -> Bus Creator/9  "<ESC_Brake_Press>"
  Bus Selector2/10 -> Bus Creator/10  "<ESC_VehSpd_Valid>"
  Bus Creator/1 -> bsVehMovInfoOut/1

== system LKAS_AutoSave_DF_20220414_1924_SW62/LKAS/LL/LLOn/LDW ==
  bsLKAInPInfo : Inport
  bsLLClb : Inport  Port=2
  Enable : EnablePort  StatesWhenEnabling=reset  ShowOutputPort=on
      settings: AttributesFormatString=states = %<StatesWhenEnabling>
  Bus Selector : BusSelector  OutputSignals=bsHdAgInfo.phiHdAg_Lft,bsHdAgInfo.phiHdAg_Rgt
  Bus Selector1 : BusSelector  OutputSignals=bsLDWClb.LL_LDWS_SUPPRESS_HEADING,bsConstantClb.LKA_SampleTime
  Cast : DataTypeConversion  OutDataTypeStr=uint8
  Heading Angle Detection (HdAgDet) : Subsystem  Description=|
      | Block Name: Heading Angle Detection
      | Ab.: HdAgDet
      | No.: 1.3.1.0
      | Rev: 0.0.1
      | Update Date: 19-3-26
  Logical Operator : Logic  Operator=NOT  AllPortsSameDT=off  OutDataTypeStr=boolean
  Product : Product  OutDataTypeStr=uint8
  LDW_Flag : Outport  OutputWhenDisabled=reset  InitialOutput=0
      settings: AttributesFormatString=%<OutputWhenDisabled> = %<InitialOutput>
  wires:
  Bus Selector1/1 -> Heading Angle Detection (HdAgDet)/4(LL_LDWS_SUPPRESS_HEADING)  "<LL_LDWS_SUPPRESS_HEADING>"
  bsLLClb/1 -> Bus Selector1/1
  Bus Selector/2 -> Heading Angle Detection (HdAgDet)/3(phiHdAg_Rgt)  "<phiHdAg_Rgt>"
  Bus Selector/1 -> Heading Angle Detection (HdAgDet)/2(phiHdAg_Lft)  "<phiHdAg_Lft>"
  Enable/1 -> Product/1, Heading Angle Detection (HdAgDet)/1(Enable)
  bsLKAInPInfo/1 -> Bus Selector/1
  Heading Angle Detection (HdAgDet)/1(stHdAgDetFlg) -> Logical Operator/1
  Product/1 -> LDW_Flag/1
  Bus Selector1/2 -> Heading Angle Detection (HdAgDet)/5(LKA_SampleTime)  "<LKA_SampleTime>"
  Cast/1 -> Product/2
  Logical Operator/1 -> Cast/1

== system LKAS_AutoSave_DF_20220414_1924_SW62/LKAS/LL/LLOn/LKA ==
  bsInInfo : Inport
  bsLKAInPInfo : Inport  Port=2
  bsLLClb : Inport  Port=3
  Enable : EnablePort  StatesWhenEnabling=reset  ShowOutputPort=on
      settings: AttributesFormatString=states = %<StatesWhenEnabling>
  Bus Selector : BusSelector  OutputSignals=bsConstantClb.LKA_SampleTime
  Cast To Single : DataTypeConversion  OutDataTypeStr=uint8
  Driver Torque Addition (DTA) : Subsystem
  LKA Exit Processing (LKAExPrcs) : Subsystem  Description=|
      | Block Name: LKA Exit Processing 
      | Ab.: LKAExPrcs
      | No.: 1.2.2.0
      | Rev: 0.0.1
      | Update Date: 19-5-13
  "LKA Motion Planning (LKAMP) " : Subsystem  Description=|
      | Block Name: LKA Motion Planning
      | Ab.: LKAMP
      | No.: 1.2.3.0
      | Rev: 0.0.1
      | Update Date: 19-5-13
  LKA SWA Limit (LKASWALim) : Subsystem  Description=|
      | Block Name: LKA SWA Synthesis
      | Ab.: LKASWASyn
      | No.: 1.2.6.0
      | Rev: 0.0.1
      | Update Date: 19-5-13
  LKA_Mon : Subsystem
  Lane Following (LF) : Subsystem  Description=|
      | Block Name: Lane Following
      | Ab.: LF
      | No.: 02
      | Rev: 00.00.01
      | Update Date: 19-3-28
  Plan To LaneFollowing (PTLF) : Subsystem
  LKA_ExitFlg : Outport  OutputWhenDisabled=reset  InitialOutput=0
      settings: AttributesFormatString=%<OutputWhenDisabled> = %<InitialOutput>
  LKA_phiSWACmd : Outport  Port=2  OutputWhenDisabled=reset  InitialOutput=0
      settings: AttributesFormatString=%<OutputWhenDisabled> = %<InitialOutput>
  LKA_M : Outport  Port=3  OutputWhenDisabled=reset  InitialOutput=0
      settings: AttributesFormatString=%<OutputWhenDisabled> = %<InitialOutput>
  LKAMon : Outport  Port=4  OutputWhenDisabled=reset  InitialOutput=0
      settings: AttributesFormatString=%<OutputWhenDisabled> = %<InitialOutput>
  tag scope: ActFlg=global, Ff=global, LKA_ExitFlg_Mon=global, LKA_SampleTime=global, PT1=global
  wires:
  [LKA_Exit3Flg] -> Driver Torque Addition (DTA)/3(DTA_Exit3Flg)
  LKA Exit Processing (LKAExPrcs)/3(LKAExPrcs_stExit3Flg) -> [LKA_Exit3Flg]
  [Ff] -> "LKA Motion Planning (LKAMP) "/2(LKAMP_Ff)
  Bus Selector/1 -> [LKA_SampleTime]  "<LKA_SampleTime>"
  [LKA_bsLLClb] -> "LKA Motion Planning (LKAMP) "/5(LKAMP_bsLLClb)
  LKA_Mon/1(LKAMon) -> LKAMon/1
  "LKA Motion Planning (LKAMP) "/2(LKAMP_tiT1) -> [PT1]  "PlanT1"
  "LKA Motion Planning (LKAMP) "/1(LKAMP_phiSWACmd) -> [Plan]  "PlanSWACmd"
  Lane Following (LF)/4(LF_phiDiffSWACmd) -> [D]
  Lane Following (LF)/2(LF_phiPropSWACmd) -> [P]
  Lane Following (LF)/1(LF_phiFfLFSWACmd) -> [Ff]
  Lane Following (LF)/3(LF_phiIntegSWACmd) -> [I]
  Driver Torque Addition (DTA)/2(DTA_M) -> LKA_M/1
  [LKAInPInfo] -> Lane Following (LF)/2(LF_bsLKAInPInfo)
  [Ff] -> LKA SWA Limit (LKASWALim)/2(LKASWALim_Ff)
  [LKA_bsInInfoSyn] -> Lane Following (LF)/1(LF_bsInInfoSyn)
  [LKA_bsInInfoSyn] -> Driver Torque Addition (DTA)/1(DTA_bsInInfoSyn)
  [LKA_bsInInfoSyn] -> "LKA Motion Planning (LKAMP) "/1(LKAMP_bsInInfoSyn)
  bsInInfo/1 -> [LKA_bsInInfoSyn]
  [LKA_bsLLClb] -> LKA SWA Limit (LKASWALim)/4(LKASWALim_bsLKAClb)
  [LKA_bsLLClb] -> Lane Following (LF)/3(LF_bsLFClb)
  [LKA_bsLLClb] -> Driver Torque Addition (DTA)/2(DTA_bsLFClb)
  [LKA_bsLLClb] -> LKA Exit Processing (LKAExPrcs)/2(LKAExPrcs_bsLKAClb)
  [LKAInPInfo] -> LKA SWA Limit (LKASWALim)/3(LKASWALim_bsLKAInPInfo)
  bsLLClb/1 -> [LKA_bsLLClb], Bus Selector/1
  [LKAInPInfo] -> Plan To LaneFollowing (PTLF)/1(InP)
  [LKAInPInfo] -> LKA Exit Processing (LKAExPrcs)/1(LKAExPrcs_bsLKAInPInfo)
  [LKAInPInfo] -> "LKA Motion Planning (LKAMP) "/4(LKAMP_bsLKAInPInfo)
  bsLKAInPInfo/1 -> [LKAInPInfo]
  [ActFlg] -> "LKA Motion Planning (LKAMP) "/3(LKAMP_stLKAActvFlg)
  [PT1] -> LKA Exit Processing (LKAExPrcs)/3(LKAExPrcs_PlanT1)
  [PT1] -> Plan To LaneFollowing (PTLF)/3(T1)
  [Plan] -> Plan To LaneFollowing (PTLF)/2(Plan)
  [DT] -> Plan To LaneFollowing (PTLF)/4(DrvTrq)
  Driver Torque Addition (DTA)/1(DTA_phiDTASWACmd) -> [DT]  "DT"
  [D] -> Plan To LaneFollowing (PTLF)/8(D)
  [I] -> Plan To LaneFollowing (PTLF)/7(I)
  [P] -> Plan To LaneFollowing (PTLF)/6(P)
  [Ff] -> Plan To LaneFollowing (PTLF)/5(Ff)
  LKA Exit Processing (LKAExPrcs)/1(LKAExPrcs_stExFlg) -> [LKA_ExitFlg_Mon], LKA_ExitFlg/1
  LKA SWA Limit (LKASWALim)/1(LKASWALim_phiSWACmd) -> LKA_phiSWACmd/1  "phiSWACmd"
  Enable/1 -> Cast To Single/1
  Plan To LaneFollowing (PTLF)/1(SWACmd) -> LKA SWA Limit (LKASWALim)/1(LKASWALim_phiTFCSWACmd)  "PTLFSWACmd"
  Cast To Single/1 -> [ActFlg]  "ActFlg"
